simulink model "controlSystem"  (R2021b)
settings: Solver=VariableStepAuto  StartTime=0.0  StopTime=10.0  RelTol=1e-3
settings Model: Creator=jcron  LastModifiedBy=jcron

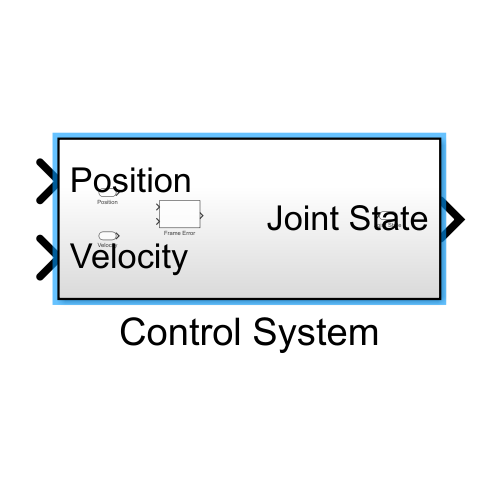
[thumbnail: Simulink's stored preview of the top-level diagram]
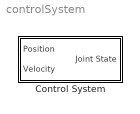
== system controlSystem ==
  Control System : Subsystem

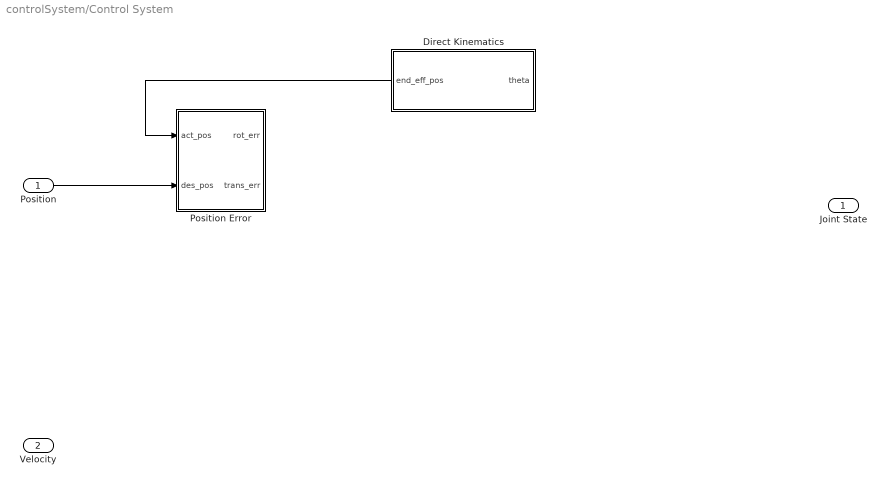
== system controlSystem/Control System ==
  Position : Inport
  Velocity : Inport  Port=2
  Direct Kinematics : MATLAB Function  TreatAsAtomicUnit=on
  Position Error : MATLAB Function  TreatAsAtomicUnit=on
  Joint State : Outport
  wires:
  Position/1 -> Position Error/2(des_pos)
  Direct Kinematics/1(end_eff_pos) -> Position Error/1(act_pos)

== matlab function controlSystem/Control System/Position Error ==
  data: act_pos input; des_pos input; rot_err output; trans_err output
function [rot_err, trans_err] = position_error(act_pos, des_pos)
desired_frame = des_pos(1:3, 1:3);
desired_origin = des_pos(1:3, 4);

actual_frame = act_pos(1:3, 1:3);
actual_origin = act_pos(1:3, 4);

trans_err = desired_origin - actual_origin;
rot_err = rotm2axang(desired_frame' * actual_frame);

== matlab function controlSystem/Control System/Direct Kinematics ==
  data: theta input; end_eff_pos output; parameters parameter
function end_eff_pos = direct_kinematics(theta, parameters)

[end_eff_frame, end_eff_origin] = direct_kinematics(theta, parameters);

end_eff_pos = [
    end_eff_frame end_eff_origin;
    zeros(1, 3) 1
];
